simulink model "NDO_STO_KDO"  (R2018a)
settings: Solver=FixedStepAuto  StartTime=0.0  StopTime=100  FixedStep=0.001  RelTol=1e-3
undefined symbols (not defined in the file or in its folder): B, k1, k2, k3, k4, k5, k6, MI
libraries: powerlib_extras x20, commchan3 x15, simulink x4, checkpacklib x1
(part 2 of 2)

== matlab function NDO_STO_KDO/ Nonlinear Observer /  ==
  data: p input; U1 input; U2 input; U3 input; U4 input; w input; x input; x_p input; uxa input; uya input; dp output; dis_z_est output; dis_x_est output; dis_y_est output; dis_fi_est output; dis_th_est output; dis_ya_est output
function [dp,dis_z_est,dis_x_est,dis_y_est,dis_fi_est,dis_th_est,dis_ya_est]= fcn(p,U1,U2,U3,U4,w,x,x_p,uxa,uya)
%%******************** parametrs *************
% m=1.83;
% Ix=21.6*10^-3;
% Iy=21.6*10^-3;
% Iz=43.2*10^-3;
% JR=3.357*10^-5;
% g=9.81;
% d=0.3;
% l=1;
xpp=x_p(1:12);
m=0.0296;
Ix=2.098*10^-5;
Iy=2.12*10^-5;
Iz=3.269*10^-5;
d=0.3;
g=9.81;
JR=(0.5*0.0025*23.1348*10^-3*23.1348*10^-3);
b=2.98*10^-5;
c=1.140*10^-7;
l=39.73*10^-3;

a1=(Iy-Iz)/Ix;
a2=-JR/Ix;
a3=(Iz-Ix)/Iy;
a4=JR/Iy;
a5=(Ix-Iy)/Iz;
b1=1/Ix;
b2=1/Iy;
b3=1/Iz;

l1=10;
l2=50;
l3=50;
l4=10;
l5=10;
l6=10;

ux=cos(x(1))*sin(x(3))*cos(x(5))+sin(x(1))*sin(x(5));
uy=cos(x(1))*sin(x(3))*sin(x(5))-sin(x(1))*cos(x(5));


%dpz=-l1*p(1)-(l1*(l1*x(7)+l2*x(8)+x(8))+l2*(-g+((1/m)*U1*(cos(x(1))*cos(x(3))))));
dpz=-l1*p(1)-l1*(l1*xpp(7)+(-g+(1/m)*U1*cos(x(1))*cos(x(3))));
%dpx=-l1*p(2)-(l1*(l1*x(9)+l2*x(10)+x(10))+l2*((uxa/m)*U1));
dpx=-l2*p(2)-l2*(l2*xpp(9)+(uxa/m)*U1);

%dpy=-l1*p(3)-(l1*(l1*x(11)+l2*x(12)+x(12))+l2*((uya/m)*U1));
dpy=-l3*p(3)-l3*(l3*xpp(11)+(uya/m)*U1);

%dprol=-l1*p(4)-(l1*(l1*x(1)+l2*x(2)+x(2))+l2*(x(4)*x(6)*a1+x(4)*a2*w+b1*U2));
dprol=-l4*p(4)-l4*(l4*xpp(1)+x(4)*x(6)*a1+x(4)*a2*w+b1*U2);

%dptheta=-l1*p(5)-(l1*(l1*x(3)+l2*x(4)+x(4))+l2*(x(2)*x(6)*a3+x(2)*a4*w+b2*U3));
dptheta=-l5*p(5)-l5*(l5*xpp(3)+x(2)*x(6)*a3+x(2)*a4*w+b2*U3);

%dpyaw=-l1*p(6)-(l1*(l1*x(5)+l2*x(6)+x(6))+l2*(x(4)*x(2)*a5+b3*U4));
dpyaw=-l6*p(6)-l6*(l6*xpp(5)+x(4)*x(2)*a5+b3*U4);


%dis_z_est=p(1)+(l1*x(7)+l2*x(8));
dis_z_est=p(1)+(l1*xpp(7));

%dis_x_est=p(2)+(l1*x(9)+l2*x(10));
dis_x_est=p(2)+(l2*xpp(9));

%dis_y_est=p(3)+(l1*x(11)+l2*x(12));
dis_y_est=p(3)+(l3*xpp(11));

%dis_fi_est=p(4)+(l1*x(1)+l2*x(2));
dis_fi_est=p(4)+(l4*xpp(1));

%dis_th_est=p(5)+(l1*x(3)+l2*x(4));
dis_th_est=p(5)+(l5*xpp(3));

%dis_ya_est=p(6)+(l1*x(5)+l2*x(6));
dis_ya_est=p(6)+(l6*xpp(5));

dp=[dpz dpx dpy dprol dptheta dpyaw];
%DT_O=[dis_z_est dis_x_est dis_y_est];
%DR_O=[dis_fi_est dis_th_est dis_ya_est];

== matlab function NDO_STO_KDO/ Kernel Differentiator Observer/MATLAB Function ==
  data: x input; x_window output; x_prev input; t input
function x_window  = fcn(x, x_prev, t)
x_window = [x_prev(2:end,:); x(1) x(3) x(5) x(7) x(9) x(11) t];

== matlab function NDO_STO_KDO/controller 2/Position controller/Position Control ==
  data: U1 output; x input; x5r input; x7r input; x7rp input; x7rpp input; x9r input; x9rp input; x9rpp input; x11r input; x11rp input; x11rpp input; DT_Z_O input; x1d output; x3d output; DT_X_O input; DT_Y_O input; uxa output; uya output
function [U1,x1d,x3d,uxa,uya] = fcn(x,x5r,x7r,x7rp,x7rpp,x9r,x9rp,x9rpp,x11r,x11rp,x11rpp,DT_Z_O,DT_X_O,DT_Y_O)
%#eml

%%%%%%%     Parametros    %%%%%%

% m=1.83;
% Ix=21.6*10^-3;
% Iy=21.6*10^-3;
% Iz=43.2*10^-3;
% d=0.3;
% g=9.81;
% JR=3.357*10^-5;
% b=2.98*10^-5;
% c=1.140*10^-7;
% l=1;

m=0.0296;
Ix=2.098*10^-5;
Iy=2.12*10^-5;
Iz=3.269*10^-5;
d=0.3;
g=9.81;
JR=(0.5*0.0025*23.1348*10^-3*23.1348*10^-3);
b=2.98*10^-5;
c=1.140*10^-7;
l=39.73*10^-3;

a1=(Iy-Iz)/Ix;
a2=-JR/Ix;
a3=(Iz-Ix)/Iy;
a4=JR/Iy;
a5=(Ix-Iy)/Iz;
b1=l/Ix;
b2=l/Iy;
b3=1/Iz;

ux=cos(x(1))*sin(x(3))*cos(x(5))+sin(x(1))*sin(x(5));
uy=cos(x(1))*sin(x(3))*sin(x(5))-sin(x(1))*cos(x(5));



%********************************************************
%                   Error para x5
%********************************************************

%k5=4;
%k6=4;

%z5=x5r-x(5);
%z6=x5rp+k5*z5-x(6);
%dz5=-k5*z5+z6;

%U4=(1/b3)*(x5rpp+k5*dz5-x(4)*x(2)*a5+k6*z6);

%********************************************************
%                   Error para x7
%********************************************************

% k7=50;
% k8=25;

k7=2.5814;
k8=0.5814;

lumda7=0.005;

% k7=1;
% k8=1;
% lumda7=1;

z7=x7r-x(7);
%s7=x7rp+k7*z7-x(8)-DT_Z_O;

s7=x7rp+k7*z7-x(8);

%z8=x7rp+k7*z7-DT_Z_O-x(8);
%dz7=-k7*z7+s7-(DT(1)-DT_Z_O);

dz7=-k7*z7+s7;

%U1=(m/(cos(x(1))*cos(x(3))))*(x7rpp+k7*dz7+z7+g+k8*z8-DT_Z_Op);

U1=(m/(cos(x(1))*cos(x(3))))*(x7rpp+k7*dz7+z7+g+k8*s7+lumda7*sign(s7)-DT_Z_O);

%U1=(m/(cos(x(1))*cos(x(3))))*(x7rpp+k7*dz7+z7+g+k8*s7+lumda7*sign(s7)-DT_Z_Op);

%********************************************************
%                   Error para x9
%********************************************************

% k9=50;
% k10=25;
% 
k9=2.5814;
k10=0.5814;

lumda9=0.0005;

% k9=200;
% k10=200;
% lumda9=1;

z9=x9r-x(9);
s10=x9rp+k9*z9-x(10);
%z10=x9rp+k9*z9-DT_X_O-x(10);
dz9=-k9*z9+s10;

%uxa=(m/(U1))*(x9rpp+k9*dz9+z9+k10*s10-DT_X_O*((z9/s10)+1)+lumda9*sign(s10));

%uxa=(m/(U1))*(x9rpp+k9*dz9+z9+k10*s10+lumda9*sign(s10)-DT_X_Op);

uxa=(m/(U1))*(x9rpp+k9*dz9+z9+k10*s10+lumda9*sign(s10)-DT_X_O);


%********************************************************
%                   Error para x11
%********************************************************

% k11=50;
% k12=25;

k11=2.5814;
k12=0.5814;

lumda11=0.0005;

% k11=200;
% k12=200;
% lumda11=1;

z11=x11r-x(11);
s12=x11rp+k11*z11-x(12);

%z12=x11rp+k11*z11-DT_Y_O-x(12);
dz11=-k11*z11+s12;


%uya=(m/(U1))*(x11rpp+k11*dz11+z11+k12*s12-DT_Y_O*((z11/s12)+1)+lumda11*sign(s12));

%uya=(m/(U1))*(x11rpp+k11*dz11+z11+k12*s12+lumda11*sign(s12)-DT_Y_Op);

uya=(m/(U1))*(x11rpp+k11*dz11+z11+k12*s12+lumda11*sign(s12)-DT_Y_O);


%%%%%%%%%%%%%%%%%%%%%%%%%%%%%%%%%%%%
%       x1d
%%%%%%%%%%%%%%%%%%%%%%%%%%%%%%%%%%%%

%x1d=sin(x(5))*uxa-cos(x(5))*uya;

x1d=sin(x5r)*uxa-cos(x5r)*uya;

%x1d=asin(comp1);

%%%%%%%%%%%%%%%%%%%%%%%%%%%%%%%%%%%%
%       x3d
%%%%%%%%%%%%%%%%%%%%%%%%%%%%%%%%%%%%

%x3d=(uxa-sin(x(1))*sin(x(5)))/(cos(x(1))*cos(x(5)));

x3d=(uxa-sin(x1d)*sin(x5r))/(cos(x1d)*cos(x5r));

%x3d=asin(comp2);

== matlab function NDO_STO_KDO/controller 2/Rotational controller /Rotational Control ==
  data: x input; x5r input; x5rp input; x5rpp input; w input; U2 output; x1d input; x1dp input; U3 output; x1dpp input; x3d input; x3dp input; x3dpp input; U4 output; DR input; DR_fi_O input; DR_th_O input; DR_ya_O input
function [U2,U3,U4] = fcn(x,x5r,x5rp,x5rpp,w,x1d,x1dp,x1dpp,x3d,x3dp,x3dpp,DR,DR_fi_O,DR_th_O,DR_ya_O)
%#eml

%%%%%%%     Parametros    %%%%%%

% m=1.83;
% Ix=21.6*10^-3;
% Iy=21.6*10^-3;
% Iz=43.2*10^-3;
% d=0.3;
% g=9.81;
% JR=3.357*10^-5;
% b=2.98*10^-5;
% c=1.140*10^-7;
% l=1;

m=0.0296;
Ix=2.098*10^-5;
Iy=2.12*10^-5;
Iz=3.269*10^-5;
d=0.3;
g=9.81;
JR=(0.5*0.0025*23.1348*10^-3*23.1348*10^-3);
b=2.98*10^-5;
c=1.140*10^-7;
l=39.73*10^-3;

a1=(Iy-Iz)/Ix;
a2=-JR/Ix;
a3=(Iz-Ix)/Iy;
a4=-JR/Iy;
a5=(Ix-Iy)/Iz;
b1=l/Ix;
b2=l/Iy;
b3=1/Iz;

ux=cos(x(1))*sin(x(3))*cos(x(5))+sin(x(1))*sin(x(5));
uy=cos(x(1))*sin(x(3))*sin(x(5))-sin(x(1))*cos(x(5));


%********************************************************
%                   Error para x1
%********************************************************

% k1=70;
% k2=40;

k1=12.8602;
k2=10.8602;

lumda1=0.001;

% k1=150;
% k2=150;
% lumda1=0.5;

z1=x1d-x(1);
s2=x1dp+k1*z1-x(2);

%z2=x1dp+k1*z1-x(2)-DR_fi_O;
dz1=-k1*z1+s2;

%U2=(1/b1)*(x1dpp+k1*dz1+z1-x(4)*x(6)*a1-x(4)*a2*w+k2*s2-DR_fi_O*((z1/s2)+1)+lumda1*sign(s2));

%U2=(1/b1)*(x1dpp+k1*dz1+z1-x(4)*x(6)*a1-x(4)*a2*w+k2*s2+lumda1*sign(s2)-DR_fi_Op);

U2=(1/b1)*(x1dpp+k1*dz1+z1-x(4)*x(6)*a1-x(4)*a2*w+k2*s2+lumda1*sign(s2)-DR_fi_O);

%********************************************************
%                   Error para x3
%********************************************************

% k3=70;
% k4=40;

k3=12.8602;
k4=10.8602;

lumda3=0.001;

% k3=150;
% k4=150;
% lumda3=0.5;

z3=x3d-x(3);
s4=x3dp+k3*z3-x(4);

%z4=x3dp+k3*z3-x(4)-DR_th_O;
dz3=-k3*z3+s4;

%U3=(1/b2)*(x3dpp+k3*dz3+z3-x(2)*x(6)*a3-x(2)*a4*w+k4*s4-DR_th_O*((z3/s4)+1)+lumda3*sign(s4));

%U3=(1/b2)*(x3dpp+k3*dz3+z3-x(2)*x(6)*a3-x(2)*a4*w+k4*s4+lumda3*sign(s4)-DR_th_Op);

U3=(1/b2)*(x3dpp+k3*dz3+z3-x(2)*x(6)*a3-x(2)*a4*w+k4*s4+lumda3*sign(s4)-DR_th_O);


%**************************************************
%                  Error para x5
%****************************************************
% k5=70;
% k6=40;
% % 
k5=12.8602;
k6=10.8602;

lumda5=0.005;

% k5=200;
% k6=200;
% lumda5=0.5;

z5=x5r-x(5);
s6=x5rp+k5*z5-x(6);

%z6=x5rp+k5*z5-x(6)+DR_ya_O;
dz5=-k5*z5+s6;

%U4=(1/b3)*(x5rpp+k5*dz5-x(4)*x(2)*a5+k6*s6-DR_ya_O*((z5/s6)+1)+lumda5*sign(s6));

%U4=(1/b3)*(x5rpp+k5*dz5+z5-x(4)*x(2)*a5+k6*s6+lumda5*sign(s6)-DR_ya_Op);

U4=(1/b3)*(x5rpp+k5*dz5+z5-x(4)*x(2)*a5+k6*s6+lumda5*sign(s6)-DR_ya_O);

== matlab function NDO_STO_KDO/ Quadrotor Plant #2/MATLAB Function1 ==
  data: disR input; DR1 output; DR2 output; DR3 output
function [DR1,DR2,DR3]= fcn(disR)

Ix=2.098*10^-5;
Iy=2.12*10^-5;
Iz=3.269*10^-5;
l=39.73*10^-3;

DR1=disR(1)/Ix;
DR2=disR(2)/Iy;
DR3=disR(3)/Iz;

== matlab function NDO_STO_KDO/ Quadrotor Plant #2/QR Plant  ==
  data: x input; w input; u input; dx_ output; DT input; DR input; uxa input; uya input
function dx_ = fcn(x,w,u,DT,DR,uxa,uya)
%#eml 

%%  PARAMETERS   (According to paper #6)%%

U=u(1:4);
% m=1.83;
% Ix=21.6*10^-3;
% Iy=21.6*10^-3;
% Iz=43.2*10^-3;
% d=0.3;
% g=9.81;
% JR=3.357*10^-5;
% b=2.98*10^-5;
% c=1.140*10^-7;
% l=1;

m=0.0296;
Ix=2.098*10^-5;
Iy=2.12*10^-5;
Iz=3.269*10^-5;
d=0.3;
g=9.81;
JR=(0.5*0.0025*23.1348*10^-3*23.1348*10^-3);
b=2.98*10^-5;
c=1.140*10^-7;
l=39.73*10^-3;

a1=(Iy-Iz)/Ix;
a2=-JR/Ix;
a3=(Iz-Ix)/Iy;
a4=-JR/Iy;
a5=(Ix-Iy)/Iz;
b1=1/Ix;
b2=1/Iy;
b3=1/Iz;

ux=cos(x(1))*sin(x(3))*cos(x(5))+sin(x(1))*sin(x(5));
uy=cos(x(1))*sin(x(3))*sin(x(5))-sin(x(1))*cos(x(5));


dx1_=x(2);
dx2_=x(4)*x(6)*a1+x(4)*a2*w+b1*U(2)+DR(1);
dx3_=x(4);
dx4_=x(2)*x(6)*a3+x(2)*a4*w+b2*U(3)+DR(2);
dx5_=x(6);
dx6_=x(4)*x(2)*a5+b3*U(4)+DR(3);
dx7_=x(8);
dx8_=-g+((1/m)*u(1)*(cos(x(1))*cos(x(3))))+DT(1);
dx9_=x(10);
dx10_=(uxa/m)*U(1)+DT(2);
dx11_=x(12);
dx12_=(uya/m)*U(1)+DT(3);
     
dx_=[dx1_ dx2_ dx3_ dx4_ dx5_ dx6_ dx7_ dx8_ dx9_ dx10_ dx11_ dx12_];

== matlab function NDO_STO_KDO/ sliding mode observer /x8 observado1 ==
  data: v2 output; v4 output; v6 output; x_ input size=[1 12]; xp input size=[1 12]; u_ input size=4; E_ input size=[1 3]; E_p output size=[1 3]; ui_ input size=[1 3]; u_p output size=[1 3]; w_ input
function [v2,v4,v6,E_p,u_p] = fcn(x_,xp,u_,E_,ui_,w_)

%********************************************
%            PLANTA BENALLEGUE   
%********************************************

%  PARAMETERS
c_c=xp(1:12);
e_e=E_(1:3);
u_k=ui_(1:3);

% m=1.83;
% Ix=21.6*10^-3;
% Iy=21.6*10^-3;
% Iz=43.2*10^-3;
% d=0.3;
% g=9.81;
% JR=3.357*10^-5;
% b=2.98*10^-5;
% c=1.140*10^-7;
% l=1;

m=0.0296;
Ix=2.098*10^-5;
Iy=2.12*10^-5;
Iz=3.269*10^-5;
d=0.3;
g=9.81;
JR=(0.5*0.0025*23.1348*10^-3*23.1348*10^-3);
b=2.98*10^-5;
c=1.140*10^-7;
l=39.73*10^-3;

a1=(Iy-Iz)/Ix;
a2=-JR/Ix;
a3=(Iz-Ix)/Iy;
a4=JR/Iy;
a5=(Ix-Iy)/Iz;
b1=l/Ix;
b2=l/Iy;
b3=1/Iz;

% m=0.468;
% Ix=4.856*10^-3;
% Iy=4.856*10^-3;
% Iz=8.801*10^-3;
% d=0.225;
% g=9.81;
% JR=3.357*10^-5;
% b=2.98*10^-5;
% c=1.140*10^-7;
% l=1;
% 
% a1=(Iy-Iz)/Ix;
% a2=-JR/Ix;
% a3=(Iz-Ix)/Iy;
% a4=-JR/Iy;
% a5=(Ix-Iy)/Iz;
% b1=l/Ix;
% b2=l/Iy;
% b3=1/Iz;


% Estimate
%%%% Perturbation z
% constant perturb
% lambda2=1000;
% alpha2=10;

% sinisoidal perturb 
lambda2=1200;
alpha2=1200;

up2=-alpha2*sign(e_e(1));

v2=-lambda2*((abs(e_e(1)))^0.5)*sign(e_e(1))+u_k(1);
x2p_est=x_(4)*x_(6)*a1+x_(4)*a2*w_+b1*u_(2)+v2;
Ep4=x2p_est-c_c(2);

% Ep1=cc(8)-x8p_est;


%%%% Perturbation x

% constant perturb
% lambda4=1000;
% alpha4=10;

% sinusoidal perturb
lambda4=1200;
alpha4=1200;

up4=-alpha4*sign(e_e(2));

v4=-lambda4*((abs(e_e(2)))^0.5)*sign(e_e(2))+u_k(2);
%fep=(cos(x(1))*sin(x(3))*cos(x(5)))+(sin(x(1))*sin(x(5)))*(1/m)*u(1);
%x10p_est=(cos(x(1))*sin(x(3))*cos(x(5)))+(sin(x(1))*sin(x(5)))*(1/m)*u(1)-af2+v10;
x4p_est=x_(2)*x_(6)*a3+x_(2)*a4*w_+b2*u_(3)+v4;

%x10p_est=fe-af2+v10;

Ep5=x4p_est-c_c(4);


%%%% Perturbation y
% sinusoidal
lambda6=1200;
alpha6=1200;

% constant
% lambda6=1000;
% alpha6=10;


up6=-alpha6*sign(e_e(3));

v6=-lambda6*((abs(e_e(3)))^0.5)*sign(e_e(3))+u_k(3);
% x12p_est=(cos(x(1))*sin(x(3))*sin(x(5)))-(sin(x(1))*cos(x(5)))*(1/m)*u(1)-af3+v12;
x6p_est=x_(4)*x_(2)*a5+b3*u_(4)+v6;

Ep6=x6p_est-c_c(6);

u_p=[up2 up4 up6];
E_p=[Ep4 Ep5 Ep6];

== matlab function NDO_STO_KDO/controller  1/Position controller/Position Control1 ==
  data: U1_ output; x_ input; x7r input; x7rp input; x7rpp input; x9r input; x9rp input; x9rpp input; x11r input; x11rp input; x11rpp input; pert_tras_ input; uxa_ output; uya_ output
function [U1_,uxa_,uya_] = fcn(x_,x7r,x7rp,x7rpp,x9r,x9rp,x9rpp,x11r,x11rp,x11rpp,pert_tras_)
%#eml

%%%%%%%     Parametros    %%%%%%
%dise_=pert_tras_(1:3);
% m=1.83;
% Ix=21.6*10^-3;
% Iy=21.6*10^-3;
% Iz=43.2*10^-3;
% d=0.3;
% g=9.81;
% JR=3.357*10^-5;
% b=2.98*10^-5;
% c=1.140*10^-7;
% l=1;

m=0.0296;
Ix=2.098*10^-5;
Iy=2.12*10^-5;
Iz=3.269*10^-5;
d=0.3;
g=9.81;
JR=(0.5*0.0025*23.1348*10^-3*23.1348*10^-3);
b=2.98*10^-5;
c=1.140*10^-7;
l=39.73*10^-3;

a1=(Iy-Iz)/Ix;
a2=-JR/Ix;
a3=(Iz-Ix)/Iy;
a4=JR/Iy;
a5=(Ix-Iy)/Iz;
b1=l/Ix;
b2=l/Iy;
b3=1/Iz;

%ux=cos(x(1))*sin(x(3))*cos(x(5))+sin(x(1))*sin(x(5));
%uy=cos(x(1))*sin(x(3))*sin(x(5))-sin(x(1))*cos(x(5));



%********************************************************
%                   Error para x5
%********************************************************

%k5=4;
%k6=4;

%z5=x5r-x(5);
%z6=x5rp+k5*z5-x(6);
%dz5=-k5*z5+z6;

%U4=(1/b3)*(x5rpp+k5*dz5-x(4)*x(2)*a5+k6*z6);

%********************************************************
%                   Error para x7
%********************************************************

k7=50;
k8=25;

% k7=2.5814;
% k8=0.5814;

lumda7=0.005;

% k7=1;
% k8=1;
% lumda7=1;

z7=x7r-x_(7);
%s7=x7rp+k7*z7-x(8)-DT_Z_O;

s7=x7rp+k7*z7-x_(8);

%z8=x7rp+k7*z7-DT_Z_O-x(8);
%dz7=-k7*z7+s7-(DT(1)-DT_Z_O);

dz7=-k7*z7+s7;

%U1=(m/(cos(x(1))*cos(x(3))))*(x7rpp+k7*dz7+z7+g+k8*z8-DT_Z_Op);

U1_=(m/(cos(x_(1))*cos(x_(3))))*(x7rpp+k7*dz7+z7+g+k8*s7+lumda7*sign(s7)-pert_tras_(1));

%U1=(m/(cos(x(1))*cos(x(3))))*(x7rpp+k7*dz7+z7+g+k8*s7+lumda7*sign(s7)-DT_Z_Op);

%********************************************************
%                   Error para x9
%********************************************************

k9=50;
k10=25;

% k9=2.5814;
% k10=0.5814;

lumda9=0.0005;

% k9=200;
% k10=200;
% lumda9=1;

z9=x9r-x_(9);
s10=x9rp+k9*z9-x_(10);
%z10=x9rp+k9*z9-DT_X_O-x(10);
dz9=-k9*z9+s10;

%uxa=(m/(U1))*(x9rpp+k9*dz9+z9+k10*s10-DT_X_O*((z9/s10)+1)+lumda9*sign(s10));

%uxa=(m/(U1))*(x9rpp+k9*dz9+z9+k10*s10+lumda9*sign(s10)-DT_X_Op);

uxa_=(m/(U1_))*(x9rpp+k9*dz9+z9+k10*s10+lumda9*sign(s10)-pert_tras_(2));


%********************************************************
%                   Error para x11
%********************************************************

k11=50;
k12=25;

% k11=2.5814;
% k12=0.5814;

lumda11=0.0005;

% k11=200;
% k12=200;
% lumda11=1;

z11=x11r-x_(11);
s12=x11rp+k11*z11-x_(12);

%z12=x11rp+k11*z11-DT_Y_O-x(12);
dz11=-k11*z11+s12;


%uya=(m/(U1))*(x11rpp+k11*dz11+z11+k12*s12-DT_Y_O*((z11/s12)+1)+lumda11*sign(s12));

%uya=(m/(U1))*(x11rpp+k11*dz11+z11+k12*s12+lumda11*sign(s12)-DT_Y_Op);

uya_=(m/(U1_))*(x11rpp+k11*dz11+z11+k12*s12+lumda11*sign(s12)-pert_tras_(3));


%%%%%%%%%%%%%%%%%%%%%%%%%%%%%%%%%%%%
%       x1d
%%%%%%%%%%%%%%%%%%%%%%%%%%%%%%%%%%%%

%x1d=sin(x(5))*uxa-cos(x(5))*uya;

%x1d=sin(x5r)*uxa-cos(x5r)*uya;

%x1d=asin(comp1);

%%%%%%%%%%%%%%%%%%%%%%%%%%%%%%%%%%%%
%       x3d
%%%%%%%%%%%%%%%%%%%%%%%%%%%%%%%%%%%%

%x3d=(uxa-sin(x(1))*sin(x(5)))/(cos(x(1))*cos(x(5)));

%x3d=(uxa-sin(x1d)*sin(x5r))/(cos(x1d)*cos(x5r));

%x3d=asin(comp2);

== matlab function NDO_STO_KDO/controller  1/ Rotational control/Rotational Control1 ==
  data: x_ input; x5r input; x5rp input; x5rpp input; w input; U2_ output; x1d input; x1dp input; U3_ output; x1dpp input; x3d input; x3dp input; x3dpp input; U4_ output; pert_rot_ input
function [U2_,U3_,U4_] = fcn(x_,x5r,x5rp,x5rpp,w,x1d,x1dp,x1dpp,x3d,x3dp,x3dpp,pert_rot_)
%#eml

%%%%%%%     Parametros    %%%%%%

% m=1.83;
% Ix=21.6*10^-3;
% Iy=21.6*10^-3;
% Iz=43.2*10^-3;
% d=0.3;
% g=9.81;
% JR=3.357*10^-5;
% b=2.98*10^-5;
% c=1.140*10^-7;
% l=1;
%dist_rot=pert_rot_(1:3);
m=0.0296;
Ix=2.098*10^-5;
Iy=2.12*10^-5;
Iz=3.269*10^-5;
d=0.3;
g=9.81;
JR=(0.5*0.0025*23.1348*10^-3*23.1348*10^-3);
b=2.98*10^-5;
c=1.140*10^-7;
l=39.73*10^-3;

a1=(Iy-Iz)/Ix;
a2=-JR/Ix;
a3=(Iz-Ix)/Iy;
a4=-JR/Iy;
a5=(Ix-Iy)/Iz;
b1=l/Ix;
b2=l/Iy;
b3=1/Iz;

%ux=cos(x(1))*sin(x(3))*cos(x(5))+sin(x(1))*sin(x(5));
%uy=cos(x(1))*sin(x(3))*sin(x(5))-sin(x(1))*cos(x(5));


%********************************************************
%                   Error para x1
%********************************************************

k1=70;
k2=40;

% k1=12.8602;
% k2=10.8602;

lumda1=0.001;

% k1=150;
% k2=150;
% lumda1=0.5;

z1=x1d-x_(1);
s2=x1dp+k1*z1-x_(2);

%z2=x1dp+k1*z1-x(2)-DR_fi_O;
dz1=-k1*z1+s2;

%U2=(1/b1)*(x1dpp+k1*dz1+z1-x(4)*x(6)*a1-x(4)*a2*w+k2*s2-DR_fi_O*((z1/s2)+1)+lumda1*sign(s2));

%U2=(1/b1)*(x1dpp+k1*dz1+z1-x(4)*x(6)*a1-x(4)*a2*w+k2*s2+lumda1*sign(s2)-DR_fi_Op);

U2_=(1/b1)*(x1dpp+k1*dz1+z1-x_(4)*x_(6)*a1-x_(4)*a2*w+k2*s2+lumda1*sign(s2)-pert_rot_(1));

%********************************************************
%                   Error para x3
%********************************************************

k3=70;
k4=40;

% k3=12.8602;
% k4=10.8602;

lumda3=0.001;

% k3=150;
% k4=150;
% lumda3=0.5;

z3=x3d-x_(3);
s4=x3dp+k3*z3-x_(4);

%z4=x3dp+k3*z3-x(4)-DR_th_O;
dz3=-k3*z3+s4;

%U3=(1/b2)*(x3dpp+k3*dz3+z3-x(2)*x(6)*a3-x(2)*a4*w+k4*s4-DR_th_O*((z3/s4)+1)+lumda3*sign(s4));

%U3=(1/b2)*(x3dpp+k3*dz3+z3-x(2)*x(6)*a3-x(2)*a4*w+k4*s4+lumda3*sign(s4)-DR_th_Op);

U3_=(1/b2)*(x3dpp+k3*dz3+z3-x_(2)*x_(6)*a3-x_(2)*a4*w+k4*s4+lumda3*sign(s4)-pert_rot_(2));


%**************************************************
%                  Error para x5
%****************************************************
k5=70;
k6=40;

% k5=12.8602;
% k6=10.8602;

lumda5=0.005;

% k5=200;
% k6=200;
% lumda5=0.5;

z5=x5r-x_(5);
s6=x5rp+k5*z5-x_(6);

%z6=x5rp+k5*z5-x(6)+DR_ya_O;
dz5=-k5*z5+s6;

%U4=(1/b3)*(x5rpp+k5*dz5-x(4)*x(2)*a5+k6*s6-DR_ya_O*((z5/s6)+1)+lumda5*sign(s6));

%U4=(1/b3)*(x5rpp+k5*dz5+z5-x(4)*x(2)*a5+k6*s6+lumda5*sign(s6)-DR_ya_Op);

U4_=(1/b3)*(x5rpp+k5*dz5+z5-x_(4)*x_(2)*a5+k6*s6+lumda5*sign(s6)-pert_rot_(3));

== matlab function NDO_STO_KDO/controller 2/Rotational controller /Rotational Control1 ==
  data: x input; x5r input; x5rp input; x5rpp input; w input; U2 output; x1d input; x1dp input; U3 output; x1dpp input; x3d input; x3dp input; x3dpp input; U4 output; DR_fi_O input; DR_th_O input; DR_ya_O input
function [U2,U3,U4] = fcn(x,x5r,x5rp,x5rpp,w,x1d,x1dp,x1dpp,x3d,x3dp,x3dpp,DR_fi_O,DR_th_O,DR_ya_O)
%#eml

%%%%%%%     Parametros    %%%%%%

% m=1.83;
% Ix=21.6*10^-3;
% Iy=21.6*10^-3;
% Iz=43.2*10^-3;
% d=0.3;
% g=9.81;
% JR=3.357*10^-5;
% b=2.98*10^-5;
% c=1.140*10^-7;
% l=1;
%dist_rot=pert_rot_(1:3);
m=0.0296;
Ix=2.098*10^-5;
Iy=2.12*10^-5;
Iz=3.269*10^-5;
d=0.3;
g=9.81;
JR=(0.5*0.0025*23.1348*10^-3*23.1348*10^-3);
b=2.98*10^-5;
c=1.140*10^-7;
l=39.73*10^-3;

a1=(Iy-Iz)/Ix;
a2=-JR/Ix;
a3=(Iz-Ix)/Iy;
a4=-JR/Iy;
a5=(Ix-Iy)/Iz;
b1=1/Ix;
b2=1/Iy;
b3=1/Iz;

ux=cos(x(1))*sin(x(3))*cos(x(5))+sin(x(1))*sin(x(5));
uy=cos(x(1))*sin(x(3))*sin(x(5))-sin(x(1))*cos(x(5));


%********************************************************
%                   Error para x1
%********************************************************

% k1=475.4068;
% k2=473.4068;

k1=68.7724;
k2=66.7724;

% k1=1.2292e03;
% k2=1.2292e03;

% k1=10;
% k2=10;

z1=x1d-x(1);
z2=x1dp+k1*z1-x(2);
dz1=-k1*z1+z2;

U2=(1/b1)*(x1dpp+k1*dz1+z1-x(4)*x(6)*a1-x(4)*a2*w+k2*z2-DR_fi_O);

%********************************************************
%                   Error para x3
%********************************************************

% k3=475.4068;
% k4=473.4068;


k3=95.8814;
k4=93.8814;

% k3=15;
% k4=12;

% k3=10;
% k4=10;

z3=x3d-x(3);
z4=x3dp+k3*z3-x(4);
dz3=-k3*z3+z4;

U3=(1/b2)*(x3dpp+k3*dz3+z3-x(2)*x(6)*a3-x(2)*a4*w+k4*z4-DR_th_O);


%**************************************************
%                  Error para x5
%****************************************************
% k5=949.8135;
% k6= 947.8135;

k5=238.2034;
k6=236.2034;

% k5=122.7473;
% k6=122.7472;

% k5=10;
% k6=10;

z5=x5r-x(5);
z6=x5rp+k5*z5-x(6);
dz5=-k5*z5+z6;

U4=(1/b3)*(x5rpp+k5*dz5+z5-x(4)*x(2)*a5+k6*z6-DR_ya_O);

== matlab function NDO_STO_KDO/controller 2/Position controller/Position Control1 ==
  data: U1 output; uxa output; uya output; x input; x5r input; x7r input; x7rp input; x7rpp input; x9r input; x9rp input; x9rpp input; x11r input; x11rp input; x11rpp input; DT_Z_O input; DT_X_O input; DT_Y_O input; x1d output; x3d output
function [U1,uxa,uya,x1d,x3d] = fcn(x,x5r,x7r,x7rp,x7rpp,x9r,x9rp,x9rpp,x11r,x11rp,x11rpp,DT_Z_O,DT_X_O,DT_Y_O)
%#eml

%%%%%%%     Parametros    %%%%%%
%dise_=pert_tras_(1:3);
% m=1.83;
% Ix=21.6*10^-3;
% Iy=21.6*10^-3;
% Iz=43.2*10^-3;
% d=0.3;
% g=9.81;
% JR=3.357*10^-5;
% b=2.98*10^-5;
% c=1.140*10^-7;
% l=1;

m=0.0296;
Ix=2.098*10^-5;
Iy=2.12*10^-5;
Iz=3.269*10^-5;
d=0.3;
g=9.81;
JR=(0.5*0.0025*23.1348*10^-3*23.1348*10^-3);
b=2.98*10^-5;
c=1.140*10^-7;
l=39.73*10^-3;

a1=(Iy-Iz)/Ix;
a2=-JR/Ix;
a3=(Iz-Ix)/Iy;
a4=JR/Iy;
a5=(Ix-Iy)/Iz;
b1=1/Ix;
b2=1/Iy;
b3=1/Iz;

%ux=cos(x(1))*sin(x(3))*cos(x(5))+sin(x(1))*sin(x(5));
%uy=cos(x(1))*sin(x(3))*sin(x(5))-sin(x(1))*cos(x(5));
%********************************************************
%                   Error para x7
%********************************************************
k7=16.8136;
k8=14.8136;

z7=x7r-x(7);
z8=x7rp+k7*z7-x(8);
dz7=-k7*z7+z8;

U1=(m/(cos(x(1))*cos(x(3))))*(x7rpp+k7*dz7+z7+g+k8*z8-DT_Z_O);

%********************************************************
%                   Error para x9
%********************************************************
k9=10.4881;
k10=8.4881;

z9=x9r-x(9);
z10=x9rp+k9*z9-x(10);
dz9=-k9*z9+z10;

uxa=(m/(U1))*(x9rpp+k9*dz9+z9+k10*z10-DT_X_O);

%********************************************************
%                   Error para x11
%********************************************************
k11=10.4881;
k12=8.4881;

z11=x11r-x(11);
z12=x11rp+k11*z11-x(12);
dz11=-k11*z11+z12;

uya=(m/(U1))*(x11rpp+k11*dz11+z11+k12*z12-DT_Y_O);

%%%%%%%%%%%%%%%%%%%%%%%%%%%%%%%%%%%%
%       x1d
%%%%%%%%%%%%%%%%%%%%%%%%%%%%%%%%%%%%
x1d=sin(x5r)*uxa-cos(x5r)*uya;
%%%%%%%%%%%%%%%%%%%%%%%%%%%%%%%%%%%%
%       x3d
%%%%%%%%%%%%%%%%%%%%%%%%%%%%%%%%%%%%
x3d=(uxa-sin(x(1))*sin(x(5)))/(cos(x(1))*cos(x(5)));

== matlab function NDO_STO_KDO/Trajectory/MATLAB Function1 ==
  data: x output; ddx output; y output; ddy output; z output; ddz output; yaw output; t input; ddyaw output; xout output
function [x,ddx,y,ddy,z,ddz,yaw,ddyaw,xout]=traj_vehic_ver1(t)

xf1=0;
yf1=0;
zf1=0;
yawf1=0; 
dxf1=0;
    dyf1=0;
    dzf1=0;
   dyawf1=0;
   ddxf1=0;
   ddyf1=0;
  ddzf1=0;
  ddyawf1=0;
if t<=5 
    
    x0=0;
    y0=0;
     z0=0;
     yaw0=0; 
     
    xf=0;
    yf=0;
    zf=1;
    yawf=0;
 tf=5;
 
a0y=y0;%yf=20;
a1y=0;
a2y=(3/(tf^2))*(yf-y0);
a3y=-(2/(tf^3))*(yf-y0);

a0x=x0;%yf=20;
a1x=0;
a2x=(3/(tf^2))*(xf-x0);
a3x=-(2/(tf^3))*(xf-x0);

a0z=z0;%zf=20;
a1z=0;
a2z=(3/(tf^2))*(zf-z0);
a3z=-(2/(tf^3))*(zf-z0);

a0yaw=yaw0;%yawf=20;
a1yaw=0;
a2yaw=(3/(tf^2))*(yawf-yaw0);
a3yaw=-(2/(tf^3))*(yawf-yaw0);

 
xf1=a0x+a2x*t^2+a3x*t^3; 
yf1=a0y+a2y*t^2+a3y*t^3;
zf1=a0z+a2z*t^2+a3z*t^3;
yawf1=a0yaw+a2yaw*t^2+a3yaw*t^3;

dxf1=2*a2x*t+3*a3x*t^2;%1.3*(pi/2.5)*sin(pi*t/2.5);%
dyf1=2*a2y*t+3*a3y*t^2;%0.5*(pi/12.5)*cos(pi*t/12.5);%
dzf1=2*a2z*t+3*a3z*t^2;
dyawf1=2*a2yaw*t+3*a3yaw*t^2;

ddxf1=2*a2x+6*a3x*t;
ddyf1=2*a2y+6*a3y*t;
ddzf1=2*a2z+6*a3z*t;
ddyawf1=2*a2yaw+6*a3yaw*t;
end

if t>5 && t<=15 
    xf1=0;
    yf1=0;
    zf1=1;
    yawf1=0;
    dxf1=0;
    dyf1=0;
    dzf1=0;
   dyawf1=0;
   ddxf1=0;
   ddyf1=0;
  ddzf1=0;
  ddyawf1=0;
end


if t>15
    
     x0=0;
     y0=0;
     z0=1;
     yaw0=0;
     
     xf=0.6;
     yf=0;
     zf=1;
     yawf=pi/4;
     
  tf=5;
a0y=y0;%yf=20;
a1y=0;
a2y=(3/(tf^2))*(yf-y0);
a3y=-(2/(tf^3))*(yf-y0);

a0x=x0;%yf=20;
a1x=0;
a2x=(3/(tf^2))*(xf-x0);
a3x=-(2/(tf^3))*(xf-x0);

a0z=z0;%yf=20;
a1z=0;
a2z=(3/(tf^2))*(zf-z0);
a3z=-(2/(tf^3))*(zf-z0);

a0yaw=yaw0;%yawf=20;
a1yaw=0;
a2yaw=(3/(tf^2))*(yawf-yaw0);
a3yaw=-(2/(tf^3))*(yawf-yaw0);
 
xf1=a0x+a2x*(t-15)^2+a3x*(t-15)^3; 
yf1=a0y+a2y*(t-15)^2+a3y*(t-15)^3;
zf1=a0z+a2z*(t-15)^2+a3z*(t-15)^3;
yawf1=a0yaw+a2yaw*(t-15)^2+a3yaw*(t-15)^3;

dxf1=2*a2x*(t-15)+3*a3x*(t-15)^2;%1.3*(pi/2.5)*sin(pi*t/2.5);%
dyf1=2*a2y*(t-15)+3*a3y*(t-15)^2;%0.5*(pi/12.5)*cos(pi*t/12.5);%
dzf1=2*a2z*(t-15)+3*a3z*(t-15)^2;
dyawf1=2*a2yaw*(t-15)+3*a3yaw*(t-15)^2;

ddxf1=2*a2x+6*a3x*(t-15);
ddyf1=2*a2y+6*a3y*(t-15);
ddzf1=2*a2z+6*a3z*(t-15);
ddyawf1=2*a2yaw+6*a3yaw*(t-15);

end

if t>20 && t<=30
     xf1=0.6;
    yf1=0;
    zf1=1;
    yawf1=pi/4;
    dxf1=0;
    dyf1=0;
    dzf1=0;
   dyawf1=0;
   ddxf1=0;
   ddyf1=0;
  ddzf1=0;
  ddyawf1=0;
end    
    if t>30
    
     x0=0.6;
     y0=0;
     z0=1;
     yaw0=pi/4;
     
     xf=0.6;
     yf=0.6;
     zf=1;
     yawf=0;
     
  tf=5;
a0y=y0;%yf=20;
a1y=0;
a2y=(3/(tf^2))*(yf-y0);
a3y=-(2/(tf^3))*(yf-y0);

a0x=x0;%yf=20;
a1x=0;
a2x=(3/(tf^2))*(xf-x0);
a3x=-(2/(tf^3))*(xf-x0);

a0z=z0;%yf=20;
a1z=0;
a2z=(3/(tf^2))*(zf-z0);
a3z=-(2/(tf^3))*(zf-z0);

a0yaw=yaw0;%yawf=20;
a1yaw=0;
a2yaw=(3/(tf^2))*(yawf-yaw0);
a3yaw=-(2/(tf^3))*(yawf-yaw0);
 
xf1=a0x+a2x*(t-30)^2+a3x*(t-30)^3; 
yf1=a0y+a2y*(t-30)^2+a3y*(t-30)^3;
zf1=a0z+a2z*(t-30)^2+a3z*(t-30)^3;
yawf1=a0yaw+a2yaw*(t-30)^2+a3yaw*(t-30)^3;

dxf1=2*a2x*(t-30)+3*a3x*(t-30)^2;%1.3*(pi/2.5)*sin(pi*t/2.5);%
dyf1=2*a2y*(t-30)+3*a3y*(t-30)^2;%0.5*(pi/12.5)*cos(pi*t/12.5);%
dzf1=2*a2z*(t-30)+3*a3z*(t-30)^2;
dyawf1=2*a2yaw*(t-30)+3*a3yaw*(t-30)^2;

ddxf1=2*a2x+6*a3x*(t-30);
ddyf1=2*a2y+6*a3y*(t-30);
ddzf1=2*a2z+6*a3z*(t-30);
ddyawf1=2*a2yaw+6*a3yaw*(t-30);
end
if t>35 && t<=45
     xf1=0.6;
    yf1=0.6;
    zf1=1;
    yawf1=0;
    dxf1=0;
    dyf1=0;
    dzf1=0;
   dyawf1=0;
   ddxf1=0;
   ddyf1=0;
  ddzf1=0;
  ddyawf1=0;
end

if t>45
    
     x0=0.6;
     y0=0.6;
     z0=1;
     yaw0=0;
     
     xf=0;
     yf=0.6;
     zf=1;
     yawf=-1/2;
     
  tf=5;
a0y=y0;%yf=20;
a1y=0;
a2y=(3/(tf^2))*(yf-y0);
a3y=-(2/(tf^3))*(yf-y0);

a0x=x0;%yf=20;
a1x=0;
a2x=(3/(tf^2))*(xf-x0);
a3x=-(2/(tf^3))*(xf-x0);

a0z=z0;%yf=20;
a1z=0;
a2z=(3/(tf^2))*(zf-z0);
a3z=-(2/(tf^3))*(zf-z0);

a0yaw=yaw0;%yawf=20;
a1yaw=0;
a2yaw=(3/(tf^2))*(yawf-yaw0);
a3yaw=-(2/(tf^3))*(yawf-yaw0);
 
xf1=a0x+a2x*(t-45)^2+a3x*(t-45)^3; 
yf1=a0y+a2y*(t-45)^2+a3y*(t-45)^3;
zf1=a0z+a2z*(t-45)^2+a3z*(t-45)^3;
yawf1=a0yaw+a2yaw*(t-45)^2+a3yaw*(t-45)^3;

dxf1=2*a2x*(t-45)+3*a3x*(t-45)^2;%1.3*(pi/2.5)*sin(pi*t/2.5);%
dyf1=2*a2y*(t-45)+3*a3y*(t-45)^2;%0.5*(pi/12.5)*cos(pi*t/12.5);%
dzf1=2*a2z*(t-45)+3*a3z*(t-45)^2;
dyawf1=2*a2yaw*(t-45)+3*a3yaw*(t-45)^2;

ddxf1=2*a2x+6*a3x*(t-45);
ddyf1=2*a2y+6*a3y*(t-45);
ddzf1=2*a2z+6*a3z*(t-45);
ddyawf1=2*a2yaw+6*a3yaw*(t-45);

end

if t>50 && t<=60
     xf1=0;
    yf1=0.6;
    zf1=1;
    yawf1=-1/2;
    dxf1=0;
    dyf1=0;
    dzf1=0;
   dyawf1=0;
   ddxf1=0;
   ddyf1=0;
  ddzf1=0;
  ddyawf1=0;
end
 if t>60
    
     x0=0;
     y0=0.6;
     z0=1;
     yaw0=-1/2;
     
     xf=0;
     yf=0;
     zf=1;
     yawf=0;
     
  tf=5;
a0y=y0;%yf=20;
a1y=0;
a2y=(3/(tf^2))*(yf-y0);
a3y=-(2/(tf^3))*(yf-y0);

a0x=x0;%yf=20;
a1x=0;
a2x=(3/(tf^2))*(xf-x0);
a3x=-(2/(tf^3))*(xf-x0);

a0z=z0;%yf=20;
a1z=0;
a2z=(3/(tf^2))*(zf-z0);
a3z=-(2/(tf^3))*(zf-z0);

a0yaw=yaw0;%yawf=20;
a1yaw=0;
a2yaw=(3/(tf^2))*(yawf-yaw0);
a3yaw=-(2/(tf^3))*(yawf-yaw0);
 
xf1=a0x+a2x*(t-60)^2+a3x*(t-60)^3; 
yf1=a0y+a2y*(t-60)^2+a3y*(t-60)^3;
zf1=a0z+a2z*(t-60)^2+a3z*(t-60)^3;
yawf1=a0yaw+a2yaw*(t-60)^2+a3yaw*(t-60)^3;

dxf1=2*a2x*(t-60)+3*a3x*(t-60)^2;%1.3*(pi/2.5)*sin(pi*t/2.5);%
dyf1=2*a2y*(t-60)+3*a3y*(t-60)^2;%0.5*(pi/12.5)*cos(pi*t/12.5);%
dzf1=2*a2z*(t-60)+3*a3z*(t-60)^2;
dyawf1=2*a2yaw*(t-60)+3*a3yaw*(t-60)^2;

ddxf1=2*a2x+6*a3x*(t-60);
ddyf1=2*a2y+6*a3y*(t-60);
ddzf1=2*a2z+6*a3z*(t-60);
ddyawf1=2*a2yaw+6*a3yaw*(t-60);
 end
if t>65 
     xf1=0;
    yf1=0;
    zf1=1;
    yawf1=0;
    dxf1=0;
    dyf1=0;
    dzf1=0;
   dyawf1=0;
   ddxf1=0;
   ddyf1=0;
  ddzf1=0;
  ddyawf1=0;
end

x=xf1;
y=yf1;
z=zf1;
yaw=yawf1;
dx=dxf1;
dy=dyf1;
dz=dzf1;
dyaw=dyawf1;
ddx=ddxf1;
ddy=ddyf1;
ddz=ddzf1;
ddyaw=ddyawf1;
xout=[xf1;yf1;zf1];

== matlab function NDO_STO_KDO/Trajectory/Valeurs désirées2/MATLAB Function ==
  data: x output; t input; y output; z output; xout output
function [x,y,z,xout]=traj_vehic(t)

xf1=0;
yf1=0;
zf1=0;
   
if t<=40 
    
    x0=0;
    y0=0;
     z0=0;
     
     
    xf=1;
    yf=2;
    
    zf=9;
 tf=40;
 
a0y=y0;%yf=20;
a1y=0;
a2y=(3/(tf^2))*(yf-y0);
a3y=-(2/(tf^3))*(yf-y0);


a0x=x0;%yf=20;
a1x=0;
a2x=(3/(tf^2))*(xf-x0);
a3x=-(2/(tf^3))*(xf-x0);


a0z=z0;%yf=20;
a1z=0;
a2z=(3/(tf^2))*(zf-z0);
a3z=-(2/(tf^3))*(zf-z0);

 
xf1=a0x+a2x*t^2+a3x*t^3;%+a4x*t^4+a5x*t^5; 
yf1=a0y+a2y*t^2+a3y*t^3;%+a4y*t^4+a5y*t^5; 
zf1=a0z+a2z*t^2+a3z*t^3;%+a4z*t^4+a5z*t^5; 

dxf=2*a2x*t+3*a3x*t^2;%1.3*(pi/2.5)*sin(pi*t/2.5);%
dyf=2*a2y*t+3*a3y*t^2;%0.5*(pi/12.5)*cos(pi*t/12.5);%
dzf=2*a2z*t+3*a3z*t^2;
end


if t>40
    
     x0=1;
     y0=2;
     z0=3;
     
     xf1=1;
     yf1=2;
     zf1=9;
    
 
end


x=xf1;
y=yf1;
z=zf1;
xout=[xf1;yf1;zf1];

== matlab function NDO_STO_KDO/MATLAB Function ==
  data: x output; dx output; ddx output; t input; y output; dy output; ddy output; z output; dz output; ddz output; yaw output
function [x,dx,ddx,y,dy,ddy,z,dz,ddz,yaw] = desired_trajectory(t)

yaw=0;
if (t>=0 && t<10)
    x=0;
    y=0;
    z=0;
   dx=0;
ddx=0;
dy=0;
ddy=0;
dz=0;
ddz=0;

else
    x=0.5*sin(2.0*pi/10.0*t);
    dx=0.5*2.0*pi/10.0*cos(2.0*pi/10.0*t);
    ddx=-0.5*2.0*pi/10.0*2.0*pi/10.0*sin(2.0*pi/10.0*t);
    
    y=0.5*cos(2.0*pi/10.0*t);
    dy=-0.5*2.0*pi/10.0*sin(2.0*pi/10.0*t);
    ddy=-0.5*2.0*pi/10.0*2.0*pi/10.0*cos(2.0*pi/10.0*t);
    z=1;
    dz=0;
    ddz=0;
    
end

== matlab function NDO_STO_KDO/ Kernel Differentiator Observer/ 1 ==
  data: U1 input; U2 input; U3 input; U4 input; uxa input; uya input; w input; x input; xp input; params input; dis_z_est output; dis_x_est output; dis_y_est output; dis_fi_est output; dis_th_est output; dis_ya_est output; params output
function [dis_z_est,dis_x_est,dis_y_est,dis_fi_est,dis_th_est,dis_ya_est, params]= fcn(U1,U2,U3,U4,uxa,uya,w,x,xp, params)

%%******************** parametrs *************
m=0.0296;
Ix=2.098*10^-5;
Iy=2.12*10^-5;
Iz=3.269*10^-5;
d=0.3;
g=9.81;
JR=(0.5*0.0025*23.1348*10^-3*23.1348*10^-3);
b=2.98*10^-5;
c=1.140*10^-7;
l=39.73*10^-3;

a1=(Iy-Iz)/Ix;
a2=-JR/Ix;
a3=(Iz-Ix)/Iy;
a4=JR/Iy;
a5=(Ix-Iy)/Iz;
b1=1/Ix;
b2=1/Iy;
b3=1/Iz;

% % If array has not been completely collected then output disturbances as
% % zero
% if x(end, 7)<25 % x(1,7)==0 &&
%     dis_z_est = 0;
%     dis_x_est = 0;
%     dis_y_est = 0; 
%     dis_fi_est = 0;
%     dis_th_est = 0;
%     dis_ya_est = 0;
%     return
% end
% 
% 
% 
% % Read the states from window
% phi_array = x(:,1); theta_array = x(:,2); psi_array = x(:,3);
% z_array = x(:,4); x_array = x(:,5); y_array = x(:,6); t_array = x(:,7);
% phi_param = params(:,1); theta_param =params(:,2); psi_param = params(:,3);
% z_param = params(:,4); x_param = params(:,5); y_param = params(:,6);
% 
% u = zeros(1,51); max_count=1000;
% %options = optimoptions('fminunc', 'MaxIterations', 20, 'UseParallel' ,true);
% 
% % Return if the latest time instant isnt a multiple of 0.025
% % This is there to reduce the number of computations
% if mod(x(end, 7), 0.025)==0
%     % Phi Estimation
%     ff = @(w)cost_func_sync_gen(w, phi_param, t_array, phi_array, u);
%     phi_param = fminsearch(ff, phi_param);
%     % theta Estimation
%     ff = @(w)cost_func_sync_gen(w, theta_param, t_array, theta_array, u);
%     theta_param = fminsearch(ff, theta_param);
%     % Psi Estimation
%     ff = @(w)cost_func_sync_gen(w, psi_param, t_array, psi_array, u);
%     psi_param = fminsearch(ff, psi_param);
%     % Z Estimation
%     ff = @(w)cost_func_sync_gen(w, z_param, t_array, z_array, u);
%     z_param = fminsearch(ff, z_param);
%     % X Estimation
%     ff = @(w)cost_func_sync_gen(w, x_param, t_array, x_array, u);
%     x_param = fminsearch(ff, x_param);
%     % Y Estimation
%     ff = @(w)cost_func_sync_gen(w, y_param, t_array, y_array, u);
%     y_param = fminsearch(ff, z_param);
% end
% 
% [phi_est_win, phi_dot_est_win, phi_ddot_est_win, ~] = output_point_estimator(t_array(end), phi_array, u, t_array(1), t_array(end), phi_param, max_count);
% [theta_est_win, theta_dot_est_win, theta_ddot_est_win, ~] = output_point_estimator(t_array(end), theta_array, u, t_array(1), t_array(end), theta_param, max_count);
% [psi_est_win, psi_dot_est_win, psi_ddot_est_win, ~] = output_point_estimator(t_array(end), psi_array, u, t_array(1), t_array(end), psi_param, max_count);
% [~, ~, z_ddot_est_win, ~] = output_point_estimator(t_array(end), z_array, u, t_array(1), t_array(end), z_param, max_count);
% [~, ~, x_ddot_est_win, ~] = output_point_estimator(t_array(end), x_array, u, t_array(1), t_array(end), x_param, max_count);
% [~, ~, y_ddot_est_win, ~] = output_point_estimator(t_array(end), y_array, u, t_array(1), t_array(end), y_param, max_count);
% 
% params = [phi_param theta_param psi_param z_param x_param y_param];
% 
% phi=phi_est_win(end); phi_dot= phi_dot_est_win(end); phi_ddot=phi_ddot_est_win(end);
% theta=theta_est_win(end); theta_dot=theta_dot_est_win(end); theta_ddot=theta_ddot_est_win(end);
% psi = psi_est_win(end); psi_dot=psi_dot_est_win(end); psi_ddot=psi_ddot_est_win(end);
% z_ddot=z_ddot_est_win(end);
% x_ddot=x_ddot_est_win(end);
% y_ddot=y_ddot_est_win(end);

xpp=xp(1:12);
phi=x(1); phi_dot= x(2); phi_ddot=xpp(2);
theta=x(3); theta_dot=x(4); theta_ddot=xpp(4);
psi = x(5); psi_dot=x(6); psi_ddot=xpp(6);
z_ddot=xpp(8);
x_ddot=xpp(10);
y_ddot=xpp(12);

% ux=cos(phi)*sin(theta)*cos(psi)+sin(phi)*sin(psi);
% uy=cos(phi)*sin(theta)*sin(psi)-sin(phi)*cos(psi);

dis_z_est = z_ddot - (-g+cos(phi)*cos(theta)*(1/m)*U1);
dis_x_est = x_ddot - ((uxa/m)*U1);
dis_y_est = y_ddot - ((uya/m)*U1);

dis_fi_est = phi_ddot - (theta_dot*psi_dot*a1 + theta_dot*a2*w + b1*U2);
dis_th_est = theta_ddot - (phi_dot*psi_dot*a3 + phi_dot*a4*w + b2*U3);
dis_ya_est = psi_ddot - (theta_dot*phi_dot*a5 + b3*U4);

% dis_z_est = 0;
% dis_x_est = 0;
% dis_y_est = 0; 
% dis_fi_est = 0;
% dis_th_est = 0;
% dis_ya_est = 0;
